simulink model "linear_model"  (R2025a)
settings: Solver=VariableStepAuto  StartTime=0.0  StopTime=10.0  RelTol=1e-3
model workspace: external: MATLAB File C:\Users\josep\Downloads\linear_model_constants.m (data not in the file)
values from neighbouring files (symbols this model uses):
  A_W = [0 1 0 ... (first row only)    [linear_model_constants.m]
  B_W = [-d_i 0 ... (first row only)    [linear_model_constants.m]
  C_W = [2/rho 0 -2]    [linear_model_constants.m]
  d_i = 0.100    (= 0.1)    [linear_model_constants.m]
  g = 9.81    [linear_model_constants.m]
settings Model: Creator=josep  LastModifiedBy=josep

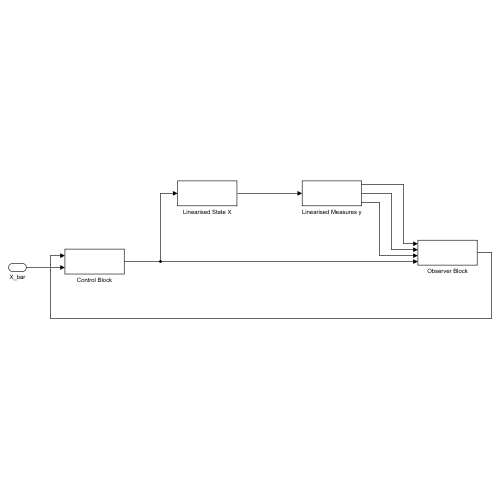
[thumbnail: Simulink's stored preview of the top-level diagram]
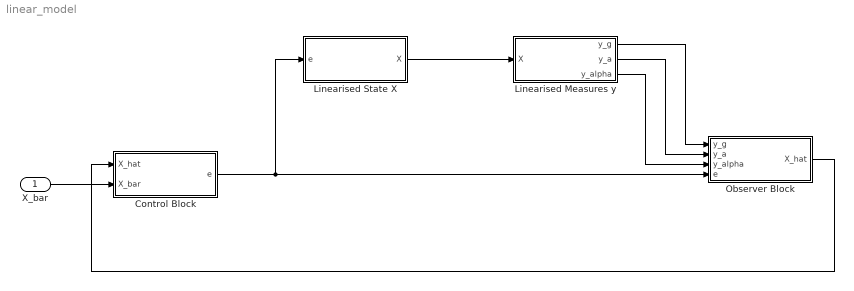
== system linear_model ==
  X_bar : Inport
  Control Block : Subsystem
  Linearised Measures y : Subsystem
  Linearised State X : Subsystem
  Observer Block : Subsystem
  wires:
  Linearised State X/1(X) -> Linearised Measures y/1(X)
  Linearised Measures y/1(y_g) -> Observer Block/1(y_g)
  Linearised Measures y/3(y_alpha) -> Observer Block/3(y_alpha)
  Linearised Measures y/2(y_a) -> Observer Block/2(y_a)
  Observer Block/1(X_hat) -> Control Block/1(X_hat)
  Control Block/1(e) -> Linearised State X/1(e), Observer Block/4(e)
  X_bar/1 -> Control Block/2(X_bar)

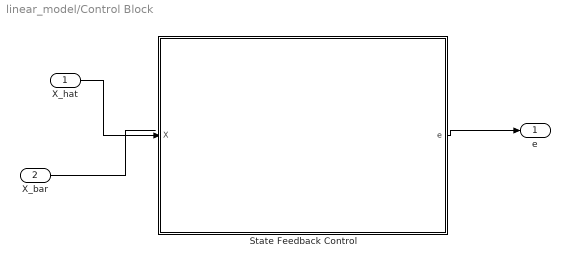
== system linear_model/Control Block ==
  X_hat : Inport
  X_bar : Inport  Port=2
  State Feedback Control : MATLAB Function  TreatAsAtomicUnit=on
  e : Outport
  wires:
  X_hat/1 -> State Feedback Control/1(X)
  X_bar/1 -> ?
  State Feedback Control/1(e) -> e/1

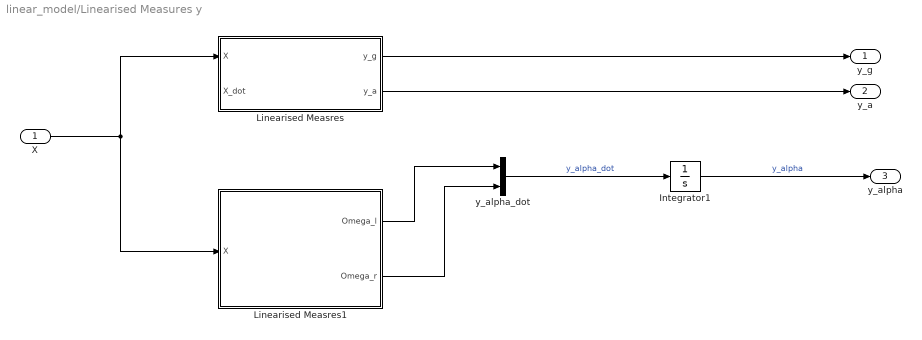
== system linear_model/Linearised Measures y ==
  X : Inport
  Integrator1 : Integrator
  Linearised Measres : MATLAB Function  TreatAsAtomicUnit=on
  Linearised Measres1 : MATLAB Function  TreatAsAtomicUnit=on
  y_alpha_dot : Mux  Inputs=2
  y_g : Outport  PortDimensions=3
  y_a : Outport  Port=2  PortDimensions=3
  y_alpha : Outport  Port=3
  wires:
  X/1 -> Linearised Measres/1(X), Linearised Measres1/1(X)
  Linearised Measres1/2(Omega_r) -> y_alpha_dot/2
  Linearised Measres1/1(Omega_l) -> y_alpha_dot/1
  Linearised Measres/2(y_a) -> y_a/1
  Linearised Measres/1(y_g) -> y_g/1
  y_alpha_dot/1 -> Integrator1/1  "y_alpha_dot"
  Integrator1/1 -> y_alpha/1  "y_alpha"

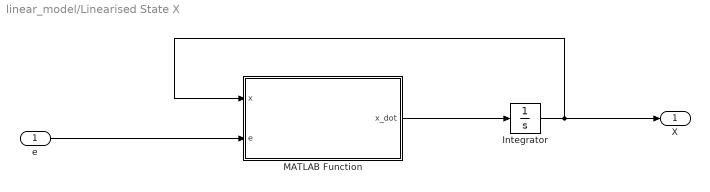
== system linear_model/Linearised State X ==
  e : Inport
  Integrator : Integrator
  MATLAB Function : MATLAB Function  TreatAsAtomicUnit=on
  X : Outport
  wires:
  e/1 -> MATLAB Function/2(e)
  MATLAB Function/1(x_dot) -> Integrator/1
  Integrator/1 -> MATLAB Function/1(x), X/1

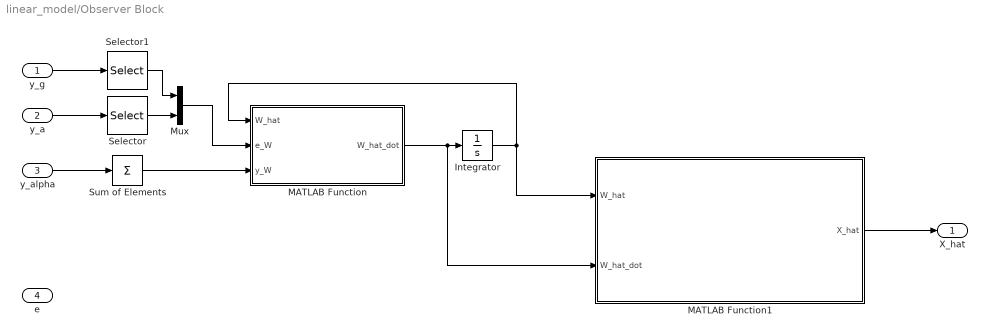
== system linear_model/Observer Block ==
  y_g : Inport
  y_a : Inport  Port=2
  y_alpha : Inport  Port=3
  e : Inport  Port=4
  Integrator : Integrator
  MATLAB Function : MATLAB Function  TreatAsAtomicUnit=on
  MATLAB Function1 : MATLAB Function  TreatAsAtomicUnit=on
  Mux : Mux  Inputs=2
  Selector : Selector  InputPortWidth=3  IndexOptions=Index vector (dialog)  Indices=1  OutputSizes=1
  Selector1 : Selector  InputPortWidth=3  IndexOptions=Index vector (dialog)  Indices=2  OutputSizes=1
  Sum of Elements : Sum  Inputs=+
  X_hat : Outport
  wires:
  MATLAB Function/1(W_hat_dot) -> MATLAB Function1/2(W_hat_dot), Integrator/1
  Integrator/1 -> MATLAB Function1/1(W_hat), MATLAB Function/1(W_hat)
  MATLAB Function1/1(X_hat) -> X_hat/1
  y_a/1 -> Selector/1
  y_g/1 -> Selector1/1
  y_alpha/1 -> Sum of Elements/1
  Sum of Elements/1 -> MATLAB Function/3(y_W)
  Selector1/1 -> Mux/1
  Selector/1 -> Mux/2
  Mux/1 -> MATLAB Function/2(e_W)

== matlab function linear_model/Linearised Measures y/Linearised Measres ==
  data: X input; y_g output; y_a output; X_dot input; g parameter; d_i parameter
function [y_g, y_a] = lin_y(X, X_dot, g, d_i)

% y_g is the 3 dimensional output that is given by C_1 X + b_1
% y_a is the 3 dimensional output, that is given by C_2 X + b_2

y_g = [0
       X(4)
       0];


y_a = [X_dot(2) - g * X(3) + d_i * X(4)
       0
       0];

== matlab function linear_model/Linearised State X/MATLAB Function ==
  data: x input; x_dot output; e input
function x_dot = lin_state_eqn(x, e)
    % e is the 2d control input dU_l and dU_r,
    % where in the cascade equation it is used as (dU_l + dU_r)
    x_dot = A * x + B * e;
end

== matlab function linear_model/Linearised Measures y/Linearised Measres1 ==
  data: X input; Omega_l output; Omega_r output; rho parameter
function [Omega_l, Omega_r] = lin_Omega(X, rho)

Omega_lr = X(2)/rho - X(4);
Omega_l = Omega_lr;
Omega_r = Omega_lr;

== matlab function linear_model/Observer Block/MATLAB Function ==
  data: W_hat input; e_W input; y_W input; W_hat_dot output; A_W parameter; C_W parameter; B_W parameter
function W_hat_dot = observer(W_hat, e_W, y_W, A_W, C_W, B_W)

% Write the observer equation out, W_hat_dot = A * W_hat + B * e + L (y -
% y_hat) where e is a 2d vector as a linear combination of y_g and y_a




y_hat = C_W * W_hat;
W_hat_dot = A_W * W_hat + B_W * e_W + L (y_W - y_hat);

== matlab function linear_model/Observer Block/MATLAB Function1 ==
  data: W_hat input; X_hat output; W_hat_dot input
function X_hat = W_hat_to_X_hat(W_hat, W_hat_dot)

X_hat = [W_hat(1)
         W_hat_dot(1)
         W_hat(3)
         W_hat_dot(3)];

== matlab function linear_model/Control Block/State Feedback Control ==
  data: X input; e output; K parameter
function e = state_feedback(X, K)
    % Function that gives the control signal for the eqn
    % X_dot = (A - BK)X + Bkr, where u = -KX + r, where r is
    % a reference consant (or non constant maybe ?)
    
    % solving the system, we get that equilibrium will be reached at x_bar =
    % - (A - BK)^-1 Br, which means that if we set a reference r, we can control
    % where the system stabilises to. Thus, r = (K - B^-1 A)x_bar
    
    % the control signal "u" here is given by the sum of components of e, so e
    % should be 
    
      e_unlimited = - K * X;
      e = [min(max(e_unlimited(1), -12), 12)
           min(max(e_unlimited(2), -12), 12)];
end
